simulink model "part3"  (R2015a)
settings: Solver=ode3  StartTime=0.0  StopTime=10  FixedStep=0.01  RelTol=1e-3
values from neighbouring files (symbols this model uses):
  K = [50; 50]    [create_data.m]
  ue = 0    [create_data.m]
  xe = [0; 0]    [create_data.m]
undefined symbols (not defined in the file or in its folder): x0
libraries: simulink x2
settings Model: Creator=vdrouinv  LastModifiedBy=vdrouinv

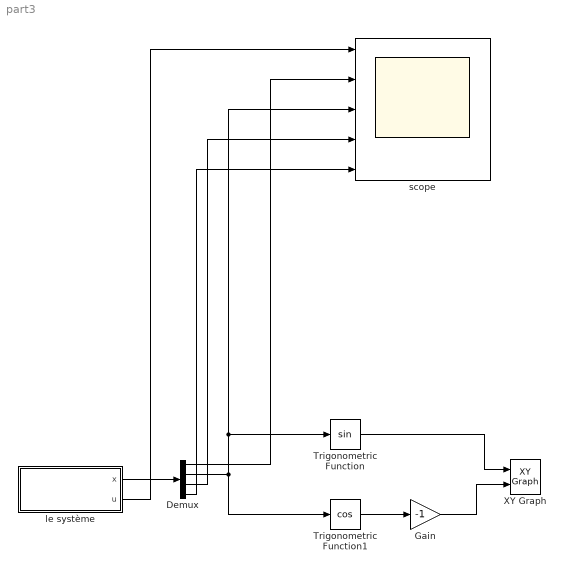
== system part3 ==
  Demux : Demux
  Gain : Gain  Gain=-1
  Trigonometric Function : Trigonometry
  Trigonometric Function1 : Trigonometry  Operator=cos
  XY Graph : simulink/Sinks/XY Graph  xmin=-1  xmax=1  ymin=-1  ymax=1  st=-1
  le système : Subsystem
  scope : Scope  NumInputPorts=5
      settings: TimeRange=10  YMin=-0.001~0.314159~-0.00175~-3.5~-0.02  YMax=0.01~0.314159~0~0.5~0.0025
  wires:
  le système/1(x) -> Demux/1
  Demux/1 -> scope/2
  Demux/3 -> scope/4
  Demux/4 -> scope/5
  le système/2(u) -> scope/1
  Trigonometric Function/1 -> XY Graph/1
  Trigonometric Function1/1 -> Gain/1
  Demux/2 -> Trigonometric Function1/1, Trigonometric Function/1, scope/3
  Gain/1 -> XY Graph/2

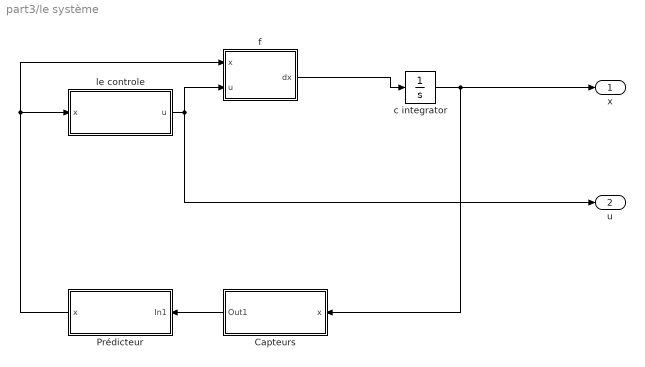
== system part3/le système ==
  Capteurs : Subsystem  TreatAsAtomicUnit=on
  Prédicteur : Subsystem  TreatAsAtomicUnit=on
  c integrator : Integrator  InitialCondition=x0
  f : MATLAB Function  TreatAsAtomicUnit=on
  le controle : Subsystem  TreatAsAtomicUnit=on
  x : Outport
  u : Outport  Port=2
  wires:
  f/1(dx) -> c integrator/1
  c integrator/1 -> x/1, Capteurs/1(x)
  le controle/1(u) -> u/1, f/2(u)
  Capteurs/1(Out1) -> Prédicteur/1(In1)
  Prédicteur/1(x) -> le controle/1(x), f/1(x)

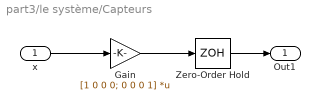
== system part3/le système/Capteurs ==
  x : Inport  PortDimensions=4
  Gain : Gain  Gain=[1 0 0 0; 0 0 0 1]  Multiplication=Matrix(K*u)
  Zero-Order Hold : ZeroOrderHold  SampleTime=0.01
  Out1 : Outport  PortDimensions=2
  wires:
  x/1 -> Gain/1
  Gain/1 -> Zero-Order Hold/1
  Zero-Order Hold/1 -> Out1/1

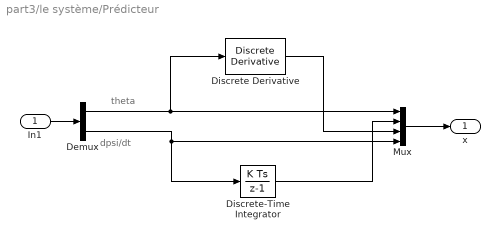
== system part3/le système/Prédicteur ==
  note: theta
  note: dpsi/dt
  In1 : Inport  PortDimensions=2
  Demux : Demux  Outputs=2
  Discrete Derivative : simulink/Discrete/Discrete Derivative  gainval=1.0  ICPrevScaledInput=0.0  InputProcessing=Inherited  OutMin=[]  OutMax=[]  OutDataType=fixdt(1, 16)  OutScaling=2^-10  DoSatur=off
  Discrete-Time Integrator : DiscreteIntegrator  InitialConditionSetting=State (most efficient)  SampleTime=-1
  Mux : Mux
  x : Outport  PortDimensions=4
  wires:
  In1/1 -> Demux/1
  Demux/1 -> Discrete Derivative/1, Mux/1
  Demux/2 -> Discrete-Time Integrator/1, Mux/4
  Mux/1 -> x/1
  Discrete Derivative/1 -> Mux/3
  Discrete-Time Integrator/1 -> Mux/2

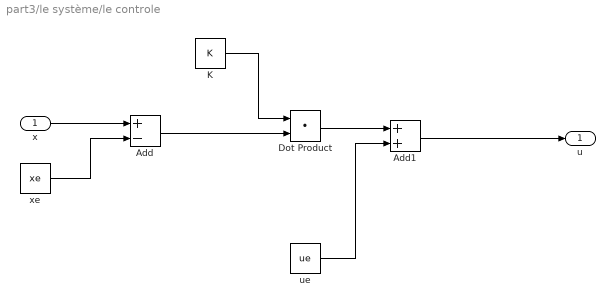
== system part3/le système/le controle ==
  x : Inport
  Add : Sum  Inputs=+-
  Add1 : Sum
  Dot Product : DotProduct  InputSameDT=on  OutDataTypeStr=Inherit: Inherit via internal rule
  K : Constant  Value=K
  ue : Constant  Value=ue
  xe : Constant  Value=xe
  u : Outport
  wires:
  x/1 -> Add/1
  xe/1 -> Add/2
  Add/1 -> Dot Product/2
  K/1 -> Dot Product/1
  Dot Product/1 -> Add1/1
  ue/1 -> Add1/2
  Add1/1 -> u/1

== matlab function part3/le système/f ==
  data: x input; u input; dx output
function dx   = f(x, u)
%   Dynamic equations of motion of the segway on an axis.
%   Inputs: - x = [theta psi dtheta dpsi]
%               theta: average angle of the wheels      [rad]
%               psi: body pitch angle                   [rad]
%               dtheta: average velocity of the wheels  [rad/s]
%               dpsi: body pitch velocity               [rad/s]
%          - u: DC motor voltage (same value for both motors) [V]

    % State
    psi = x(2);
    dtheta = x(3);
    dpsi = x(4);

    % Parameters
    
    g = 9.81;           % gravity acceleration [m/sec^2]
    m = 0.03;           % wheel weight [kg]
    R = 0.04;           % wheel radius [m]
    Jw = m*R^2/2;       % wheel inertia moment [kg*m^2]
    M = 0.6;            % body weight [kg]
    H = 0.144;          % body height [m]
    L = H/2;            % distance of the center of mass from the wheel axle [m]
    Jpsi = M*L^2/3;     % body pitch inertia [kgm^2]
    Jm = 1e-5;          % DC motor inertia moment [kgm^2]
    Rm = 6.69;          % DC motor resistance [Ohm]
    Kb = 0.468;         % DC motor back EMF constant [Vsec/rad]
    Kt = 0.317;         % DC motor torque constant [Nm/A]
    n = 1;              % gear ratio
    fm = 0.0022;        % friction coefficient between body and DC motor
    fw = 0;             % friction coefficient between wheel and floor
    
    % Equations of motion
    c1 = (2*m+M)*R^2 + 2*Jw + 2*n^2*Jm;
    c2 = M*L*R*cos(psi) - 2*n^2*Jm;
    c3 = -M*L*R*dpsi^2*sin(psi);
    c4 = M*L^2 + Jpsi + 2*n^2*Jm;
    c5 = -M*g*L*sin(psi);

    alpha = Kt/Rm;
    beta = Kt*Kb/Rm + fm;

    Ftheta = alpha*(2*u) - 2*(beta+fw)*dtheta + 2*beta*dpsi;
    Fpsi = -alpha*(2*u) + 2*beta*dtheta - 2*beta*dpsi;

    ddtheta = (c4*c3 - c2*c5 + c4*Ftheta - c2*Fpsi)/(c4*c1 - c2^2);
    ddpsi = (Fpsi- c2*ddtheta - c5)/c4;
    dx = [dtheta dpsi ddtheta ddpsi]';

end

% Matrices of the linearized system
% E = [(2*m+M)*R^2+2*Jw+2*Jm   M*L*R-2*Jm; M*L*R-2*Jm   M*L^2+Jpsi+2*Jm];
% detE = det(E);

% alpha = Kt/Rm;
% beta = Kt*Kb/Rm + fm;

% A32 = -M*g*L*E(1,2)/detE;
% A42 = M*g*L*E(1,1)/detE;
% A33 = -(beta*E(2,2)+2*beta*E(1,2))/detE;
% A43 = (beta*E(1,2)+2*beta*E(1,1))/detE;
% A34 = beta*(E(2,2)+2*E(1,2))/detE;
% A44 = -beta*(E(1,2)+2*E(1,1))/detE;

% B3 = alpha*(E(2,2)/2+E(1,2))/detE;
% B4 = -alpha*(E(1,2)/2+E(1,1))/detE;

% A = [0 0 1 0;0 0 0 1; 0 A32 A33 A34; 0 A42 A43 A44];
% B = [0 0 2*B3 2*B4];
